simulink model "AudioSmartSpeakerOnJetsonNano"  (R2026a)
settings: Solver=FixedStepAuto  StopTime=inf  EnableMultiTasking=on
InitFcn:
  | initializeAudioSmartSpeakerOnRaspiModelParameters;
values from neighbouring files (symbols this model uses):
  frameLengthSpeech = windowDuration*speechFs    (= 1600)    [initializeAudioSmartSpeakerOnRaspiModelParameters.m]
  windowDuration = 0.1    [initializeAudioSmartSpeakerOnRaspiModelParameters.m]
undefined symbols (not defined in the file or in its folder): plughw
libraries: nvidiaAVlib x7, audiofilters x2, dspsigops x1, audiodynamicrange x1, audiofeatures x1, deeplib x1, dspmathops x1
settings Model: ExtModeTrigDuration=2  Creator=The MathWorks, Inc.  LastModifiedBy=KoayXianCong
settings SolverCC: PositivePriorityOrder=on
settings OptimizationCC: MaxStackSize=200000  SimCompilerOptimization=on
settings DebuggingCC: AlgebraicLoopMsg=error  SingleTaskRateTransMsg=error  IntegerOverflowMsg=none  ParameterPrecisionLossMsg=none  IntegerSaturationMsg=none
settings HardwareCC: ProdBitPerLong=64.0  ProdLargestAtomicInteger=LongLong  ProdLargestAtomicFloat=Double  ProdHWDeviceType=ARM Compatible->ARM Cortex-A (64-bit)
settings ModelReferenceCC: PropagateVarSize=During execution
settings SFSimCC: SimCtrlC=off
settings RTWCC: SystemTargetFile=ert.tlc  HardwareBoard=NVIDIA Jetson  TLCOptions="-aInlineSetEventsForThisBaseRateFcn=TLC_FALSE -aSuppressMultiTaskScheduler=TLC_FALSE  -aRateBasedStepFcn=0"  CustomDefine=_GNU_SOURCE  BuildConfiguration=Faster Runs  DLArmComputeArch=armv7  Description=Embedded Coder
settings CodeAppCC: MaxIdLength=100.0
settings ERTTargetCC: ExtModeTransport=2.0  RootIOFormat=Structure reference  CodeReplacementLibrary=ARM Cortex-A CMSIS  SupportContinuousTime=on  SupportVariableSizeSignals=on
settings SimscapeCC: SimscapeNominalValues="[{\"value\":\"1\",\"unit\":\"A\"},{\"value\":\"1\",\"unit\":\"bar\"},{\"value\":\"1\",\"unit\":\"cm^2\"},{\"value\":\"1\",\"unit\":\"cm^3/s\"},{\"value\":\"1\",\"unit\":\"kJ/kg\"},{\"value\":\"1\",\"unit\":\"kW\"},{\"value\":\"1\",\"unit\":\"l\"},{\"value\":\"1\",\"unit\":\"N\"},{\"value\":\"1\",\"unit\":\"N*m\"},{\"value\":\"1\",\"unit\":\"V\"}]"  SimscapeLogType=none  SimscapeLogDataHistory=5000.0

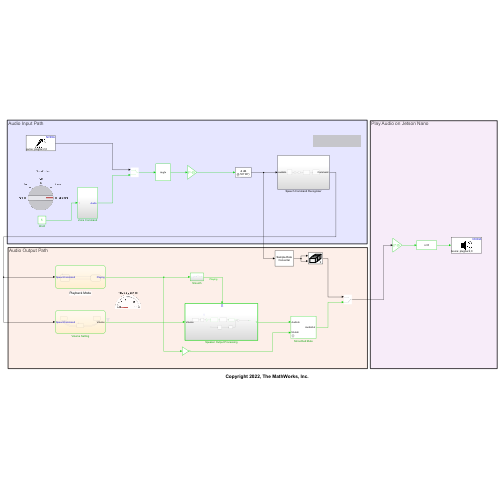
[thumbnail: Simulink's stored preview of the top-level diagram]
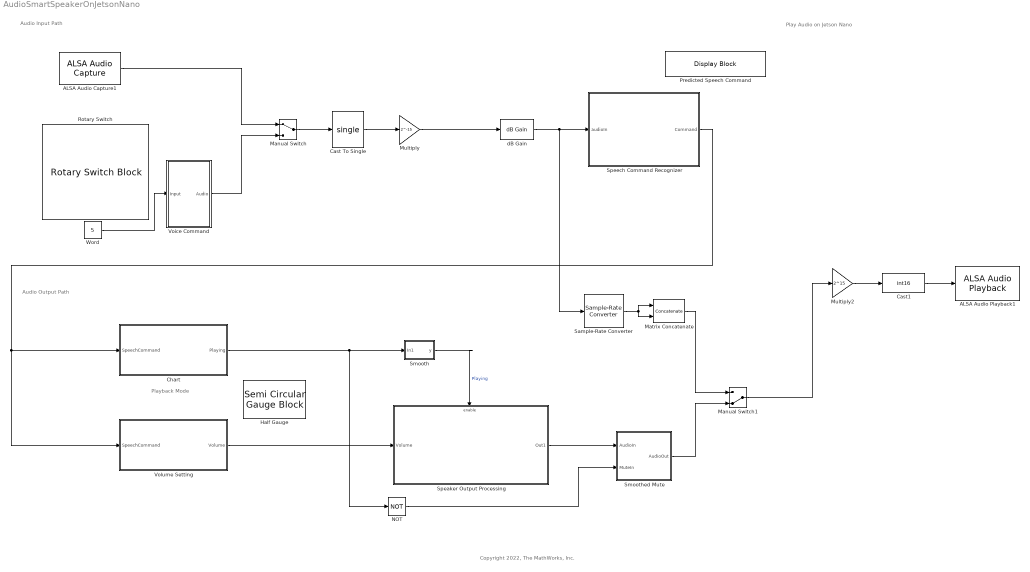
== system AudioSmartSpeakerOnJetsonNano ==
  note: Play Audio on Jetson Nano
  note: Audio Output Path
  note: Audio Input Path
  note: Copyright 2022, The MathWorks, Inc.
  note: Playback Mode
  ALSA Audio Capture1 : nvidiaAVlib/ALSA Audio Capture  deviceStr=plughw:2,0  DataBitDepth=16-bit integer  numberOfChannels=1  sampleRateEnum=16000  frameSize=frameLengthSpeech  QueueDuration=0.5  blockPlatform=LINUX
  ALSA Audio Playback1 : nvidiaAVlib/ALSA Audio Playback  deviceStr=plughw:2,0  sampleRateEnum=44100  queueDuration=0.5  blockPlatform=LINUX
  Cast To Single : DataTypeConversion  OutDataTypeStr=single  SaturateOnIntegerOverflow=off  RndMeth=Floor
  Cast1 : DataTypeConversion  OutDataTypeStr=int16  SaturateOnIntegerOverflow=off  RndMeth=Floor
  Chart : Stateflow chart  TreatAsAtomicUnit=on  SystemSampleTime=windowDuration
  Half Gauge : SemiCircularGaugeBlock  ScaleMax=15  FontColor=[0.0, 0.0, 0.0]
  Manual Switch : ManualSwitch
  Manual Switch1 : ManualSwitch  CurrentSetting=0
  Matrix Concatenate : Concatenate  Mode=Multidimensional array  ConcatenateDimension=2
  Multiply : Gain  Gain=2^-15
  Multiply2 : Gain  Gain=2^15
  NOT : Logic  Operator=NOT  IconShape=distinctive  AllPortsSameDT=off  OutDataTypeStr=boolean
  Predicted Speech Command : DisplayBlock  LabelPosition=Hide  GridColor=[0.502, 0.502, 0.502]
  Rotary Switch : RotarySwitchBlock
  Sample-Rate Converter : dspsigops/Sample-Rate Converter  InputSampleRate=16000  OutputSampleRate=44100  OutputRateTolerance=0  Bandwidth=12000  StopbandAttenuation=80  AllowArbitraryInputLength=off  SimulateUsing=Code generation
  Smooth : Subsystem
  Smoothed Mute : Subsystem  mask{tau=0.396}
  "Speaker Output Processing " : Subsystem  TreatAsAtomicUnit=on
  Speech Command Recognizer : Subsystem
  Voice Command : Subsystem
  Volume Setting : Stateflow chart  TreatAsAtomicUnit=on  SystemSampleTime=windowDuration
  Word : Constant  Value=5  SampleTime=0.1
  dB Gain : dspmathops/dB Gain  dB=-6  intype=Amplitude
  wires:
  Cast To Single/1 -> Multiply/1
  ALSA Audio Capture1/1 -> Manual Switch/1
  Manual Switch/1 -> Cast To Single/1
  Word/1 -> Voice Command/1(Input)
  Voice Command/1(Audio) -> Manual Switch/2
  Multiply/1 -> dB Gain/1
  dB Gain/1 -> Sample-Rate Converter/1, Speech Command Recognizer/1(audioIn)
  NOT/1 -> Smoothed Mute/2(MuteIn)
  Smooth/1(y) -> "Speaker Output Processing "/Enable  "Playing"
  "Speaker Output Processing "/1(Out1) -> Smoothed Mute/1(AudioIn)
  Chart/1(" Playing") -> NOT/1, Smooth/1(In1)
  Volume Setting/1(Volume) -> "Speaker Output Processing "/1(Volume)
  Speech Command Recognizer/1(Command) -> Chart/1(SpeechCommand), Volume Setting/1(SpeechCommand)
  Matrix Concatenate/1 -> Manual Switch1/1
  Sample-Rate Converter/1 -> Matrix Concatenate/1, Matrix Concatenate/2
  Multiply2/1 -> Cast1/1
  Cast1/1 -> ALSA Audio Playback1/1
  Smoothed Mute/1(AudioOut) -> Manual Switch1/2
  Manual Switch1/1 -> Multiply2/1

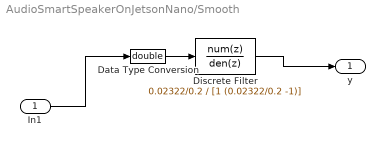
== system AudioSmartSpeakerOnJetsonNano/Smooth ==
  In1 : Inport
  Data Type Conversion : DataTypeConversion  OutDataTypeStr=double  SaturateOnIntegerOverflow=off  RndMeth=Floor
  Discrete Filter : DiscreteFilter  Numerator=0.02322/0.2  Denominator=[1 (0.02322/0.2 -1)]  InputProcessing=Columns as channels (frame based)
  y : Outport
  wires:
  Data Type Conversion/1 -> Discrete Filter/1
  In1/1 -> Data Type Conversion/1
  Discrete Filter/1 -> y/1

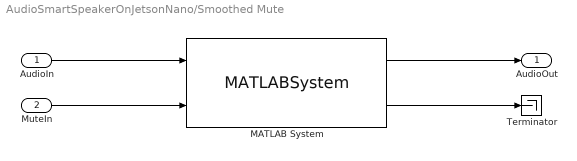
== system AudioSmartSpeakerOnJetsonNano/Smoothed Mute ==
  AudioIn : Inport
  MuteIn : Inport  Port=2  SampleTime=windowDuration
  MATLAB System : MATLABSystem  System=SmoothedMute  Tau=tau  SampleRate=44100  SimulateUsing=Code generation
      mask Type: SmoothedMute
  Terminator : Terminator
  AudioOut : Outport  VectorParamsAs1DForOutWhenUnconnected=off
  wires:
  MuteIn/1 -> MATLAB System/2
  MATLAB System/2 -> Terminator/1
  MATLAB System/1 -> AudioOut/1
  AudioIn/1 -> MATLAB System/1

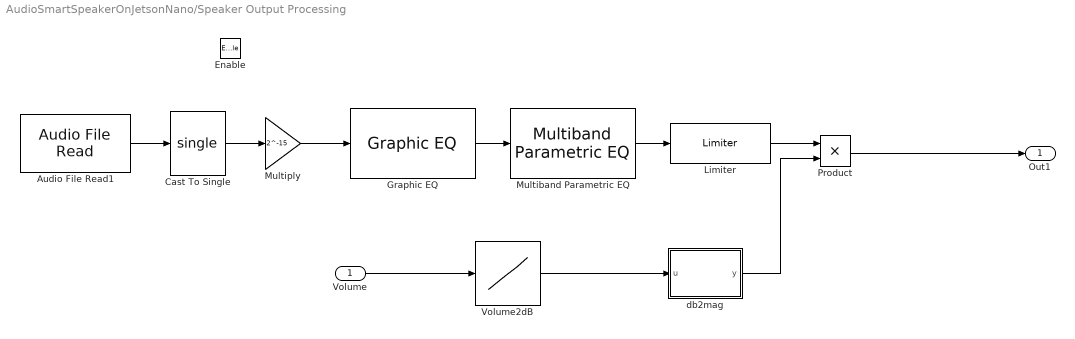
== system AudioSmartSpeakerOnJetsonNano/Speaker Output Processing  ==
  Volume : Inport
  Enable : EnablePort
  Audio File Read1 : nvidiaAVlib/Audio File Read  FileName=RockGuitar-16-44p1-stereo-72secs.wav  PlayCount=Inf  OutputEOFIndicator=off  SamplesPerFrame=4410
  Cast To Single : DataTypeConversion  OutDataTypeStr=single  SaturateOnIntegerOverflow=off  RndMeth=Floor
  Graphic EQ : audiofilters/Graphic EQ  EQOrder=2  Bandwidth=1 octave  Structure=Cascade  Gain_25=0  Gain_31_5=-4.0  Gain_40=0  Gain_50=0  Gain_63=0  Gain_80=0  Gain_100=0  Gain_125=5.200  Gain_160=0  Gain_200=0  Gain_250=-6.0  Gain_315=0  Gain_400=0  Gain_500=6.800  Gain_630=0  Gain_800=0  Gain_1000=-2.0  Gain_1250=0  Gain_1600=0  Gain_2000=-1.200  Gain_2500=0  Gain_3150=0  Gain_4000=0  Gain_5000=0  Gain_6300=0  Gain_8000=0.400  Gain_10000=0  Gain_12500=0  Gain_16000=0  Gain_20000=0  WorkspaceVariableName=myFilt  OverwriteExportVariable=on  InheritSampleRate=off  SampleRate=44100  SimulateUsing=Code generation
  Limiter : audiodynamicrange/Limiter  ThresholdPort=off  Threshold=-6.500  KneeWidthPort=off  KneeWidth=0.0  AttackTimePort=off  AttackTime=0.0  ReleaseTimePort=off  ReleaseTime=0.2  MakeUpGainMode=Property  MakeUpGain=0.0  InheritSampleRate=on  SampleRate=44100  outputGain=off  EnableSidechain=off  SimulateUsing=Code generation
  Multiband Parametric EQ : audiofilters/Multiband Parametric EQ  EQOrder=2  NumEQBands=3  FrequenciesPort=off  Frequencies=[100 1000 5000]  PeakGainsPort=off  PeakGains=[0 0 0]  QualityFactorsPort=off  QualityFactors=[1.6 1.6 1.6]  InheritSampleRate=off  SampleRate=44100  WorkspaceVariableName=myFilt  OverwriteExportVariable=on  HasLowShelfFilter=off  LowShelfCutoffPort=off  LowShelfCutoff=200  LowShelfSlopePort=off  LowShelfSlope=1.5  LowShelfGainPort=off  LowShelfGain=0  HasHighShelfFilter=off  HighShelfCutoffPort=off  HighShelfCutoff=15e3  HighShelfSlopePort=off  HighShelfSlope=1.5  HighShelfGainPort=off  HighShelfGain=0  HasLowpassFilter=off  LowpassCutoffPort=off  LowpassCutoff=18e3  LowpassSlopePort=off  LowpassSlope=12  HasHighpassFilter=off  HighpassCutoffPort=off  HighpassCutoff=20  HighpassSlopePort=off  HighpassSlope=30  Oversample=off  SimulateUsing=Code generation
  Multiply : Gain  Gain=2^-15  OutDataTypeStr=Inherit: Same as input
  Product : Product
  Volume2dB : Lookup_n-D  NumberOfTableDimensions=1  BreakpointsForDimension1=[1:12]  Table=[-70,-60,-50,-40,-35,-30,-25,-20,-15,-10,-5,0]  InternalRulePriority=Speed  RndMeth=Simplest
  db2mag : MATLAB Function  TreatAsAtomicUnit=on
  Out1 : Outport
  wires:
  Limiter/1 -> Product/1
  Product/1 -> Out1/1
  Graphic EQ/1 -> Multiband Parametric EQ/1
  Multiband Parametric EQ/1 -> Limiter/1
  Volume/1 -> Volume2dB/1
  Volume2dB/1 -> db2mag/1(u)
  db2mag/1(y) -> Product/2
  Audio File Read1/1 -> Cast To Single/1
  Cast To Single/1 -> Multiply/1
  Multiply/1 -> Graphic EQ/1

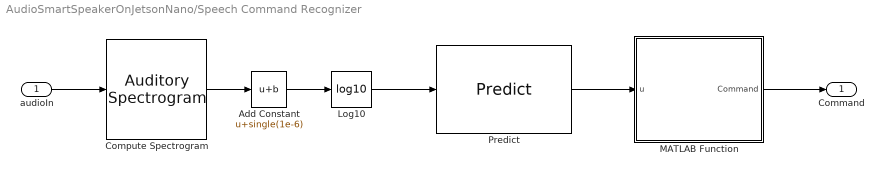
== system AudioSmartSpeakerOnJetsonNano/Speech Command Recognizer ==
  audioIn : Inport
  Add Constant : Bias  Bias=single(1e-6)  SaturateOnIntegerOverflow=off
  Compute Spectrogram : audiofeatures/Auditory Spectrogram  FrequencyScale=bark  MelStyle=oshaughnessy  AutoNumBands=off  NumBands=50  AutoFrequencyRange=on  FrequencyRange=[0, 22050]  FilterBankDesignDomain=linear  FilterBankNormalization=bandwidth  OutputFrequencyVector=off  WindowParameter="hann(round(0.025*16e3),\"periodic\")"  WindowNormalization=off  OverlapLength=round(0.015*16e3)  AutoFFTLength=off  FFTLength=512  SpectrumType=power  ApplyLog=off  NumHops=98  NumHopsOverlap=88  InheritSampleRate=off  SampleRate=16e3
  Log10 : Math  Operator=log10
  MATLAB Function : MATLAB Function  TreatAsAtomicUnit=on
  Predict : deeplib/Predict  Network=Network from MAT-file  NetworkFunction=squeezenet  NetworkFilePath=PrunedSpeechCommandRecognitionNetwork.mat  MiniBatchSize=128  SimulateUsing=Auto mode  InputDataFormats={'imageinput', 'SSCB';}  Predictions=on  Activations={}  ForceInterpretedSim=off  EnableDLNetwork=on  LastKnownNetworkFilePath='PrunedSpeechCommandRecognitionNetwork.mat'  LastKnownNetworkTimeStamp=740102.371886574081145226955413818359375
  Command : Outport
  wires:
  Log10/1 -> Predict/1
  audioIn/1 -> Compute Spectrogram/1
  Predict/1 -> MATLAB Function/1(u)
  Compute Spectrogram/1 -> Add Constant/1
  Add Constant/1 -> Log10/1
  MATLAB Function/1(Command) -> Command/1

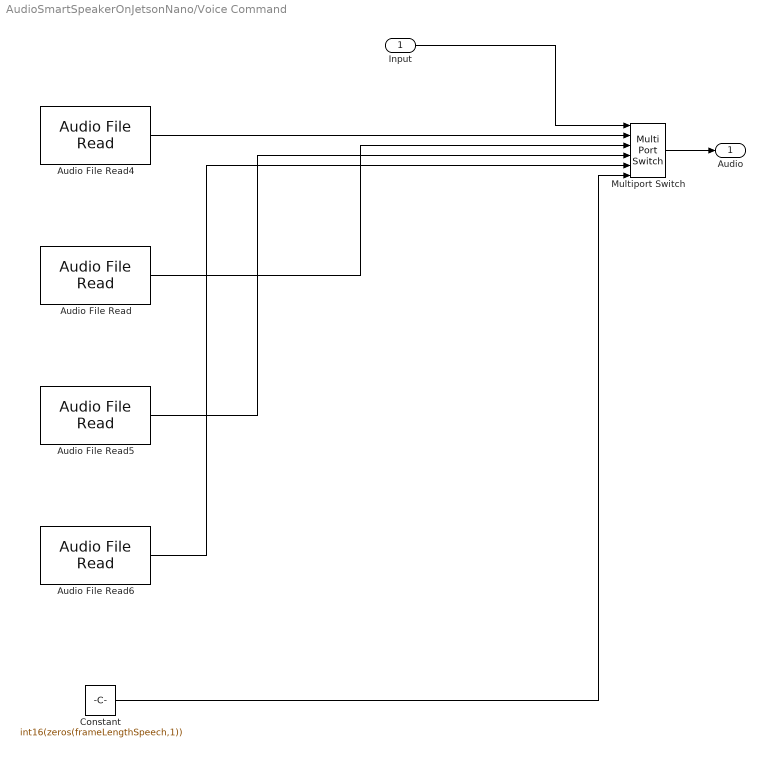
== system AudioSmartSpeakerOnJetsonNano/Voice Command ==
  Input : Inport
  Audio File Read : nvidiaAVlib/Audio File Read  FileName=stop.wav  PlayCount=Inf  OutputEOFIndicator=off  SamplesPerFrame=frameLengthSpeech
  Audio File Read4 : nvidiaAVlib/Audio File Read  FileName=go.wav  PlayCount=Inf  OutputEOFIndicator=off  SamplesPerFrame=frameLengthSpeech
  Audio File Read5 : nvidiaAVlib/Audio File Read  FileName=up.wav  PlayCount=Inf  OutputEOFIndicator=off  SamplesPerFrame=frameLengthSpeech
  Audio File Read6 : nvidiaAVlib/Audio File Read  FileName=down.wav  PlayCount=Inf  OutputEOFIndicator=off  SamplesPerFrame=frameLengthSpeech
  Constant : Constant  Value=int16(zeros(frameLengthSpeech,1))  OutDataTypeStr=int16  SampleTime=0.1
  Multiport Switch : MultiPortSwitch  Inputs=5  SaturateOnIntegerOverflow=off  InputSameDT=off
  Audio : Outport  VectorParamsAs1DForOutWhenUnconnected=off
  wires:
  Audio File Read4/1 -> Multiport Switch/2
  Input/1 -> Multiport Switch/1
  Audio File Read/1 -> Multiport Switch/3
  Audio File Read5/1 -> Multiport Switch/4
  Audio File Read6/1 -> Multiport Switch/5
  Constant/1 -> Multiport Switch/6
  Multiport Switch/1 -> Audio/1

== stateflow chart AudioSmartSpeakerOnJetsonNano/Chart ==
  state Off
  state Playing
  (default) -> Off
  Off -> Playing : [SpeechCommand == SpeechCommands.Go]
  Playing -> Off : [SpeechCommand == SpeechCommands.Stop]
  data: SpeechCommand input Enum: SpeechCommands; Playing output boolean

== matlab function AudioSmartSpeakerOnJetsonNano/Speaker Output Processing /db2mag ==
  data: u input; y output
function y = fcn(u)

y = 1/db2mag(abs(u));

== stateflow chart AudioSmartSpeakerOnJetsonNano/Volume Setting ==
  state DecrementVolume
    en:Volume = Volume-1
  state IncrementVolume
    en:Volume = Volume+1
  state VolumeSteady
  DecrementVolume -> VolumeSteady : after(40,tick)
  VolumeSteady -> DecrementVolume [order 1] : [SpeechCommand == SpeechCommands.Down]
  IncrementVolume -> VolumeSteady : after(40,tick)
  VolumeSteady -> IncrementVolume [order 2] : [SpeechCommand == SpeechCommands.Up]
  (default) -> VolumeSteady
  data: SpeechCommand input Enum: SpeechCommands; Volume output =6

== matlab function AudioSmartSpeakerOnJetsonNano/Speech Command Recognizer/MATLAB Function ==
  data: u input; Command output size=[1 1]
function Command = postProcess(u)
    
    classificationRate = 10;
    persistent YBuffer probBuffer
    
    if(isempty(YBuffer))
        YBuffer = ones(classificationRate,1);
        probBuffer = zeros([numel(u),round(classificationRate/2)]);
    end
    
    % Input u is array of 12 probability values (which word was most likely
    % to be spoken)

    % Find index of array with highest probability and enumerate to our
    % word
    [~,YPredicted] = max(u);
    
    % Add to buffers
    YBuffer(1:end-1)= YBuffer(2:end);
    YBuffer(end) = YPredicted;
    probBuffer(:,1:end-1) = probBuffer(:,2:end);
    probBuffer(:,end) = u;
    
    % Now do the actual command detection by performing a very simple
    % thresholding operation. Declare a detection and display it 
    % if all of the following hold:
    % 1) The most common label is not |background|.
    % 2) At least |countThreshold| of the latest frame labels agree.
    % 3) The maximum predicted probability of the predicted label is at
    % least |probThreshold|. Otherwise, do not declare a detection.

    [YMode,count] = mode(YBuffer,1);
    countThreshold = ceil(classificationRate*0.2);
    maxProb = max(probBuffer(YMode,:));
    probThreshold = 0.5;

    if (count > countThreshold && maxProb > probThreshold && YMode ~= SpeechCommands.Background)
        Command = SpeechCommands(YMode);
    else
        Command = SpeechCommands(0);
    end
    
end
